simulink model "untitled"  (R2023b)
settings: Solver=VariableStepAuto  StartTime=0.0  StopTime=20  RelTol=1e-3
undefined symbols (not defined in the file): tdead, Vth
libraries: spsMosfetLib x8, spsCurrentMeasurementLib x2, spsParallelRLCBranchLib x2, simulink x2, spsLinearTransformerLib x1, spsDCVoltageSourceLib x1, slpidlib x1, spsSeriesRLCBranchLib x1, spsVoltageMeasurementLib x1, spspowerguiLib x1
settings Model: Creator=Dell  LastModifiedBy=Dell

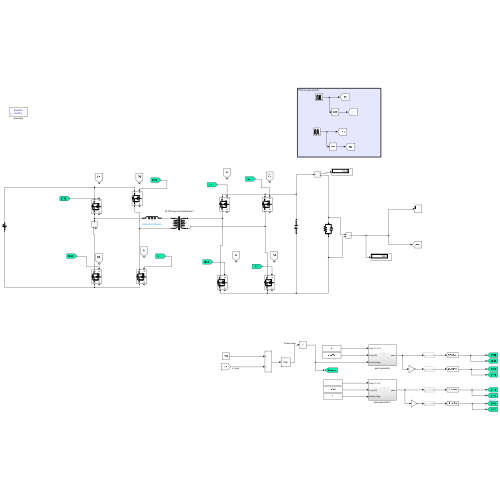
[thumbnail: Simulink's stored preview of the top-level diagram]
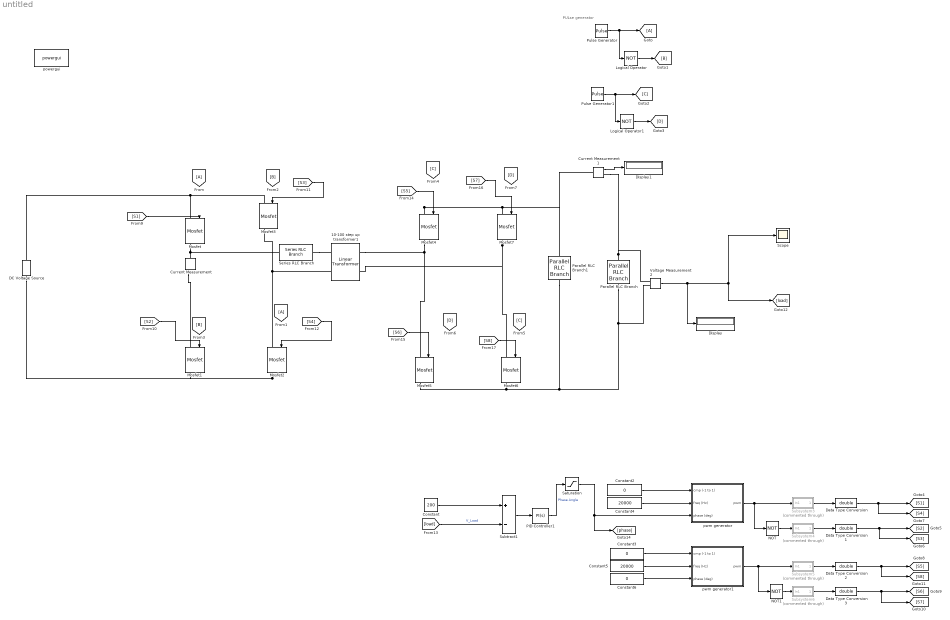
== system untitled ==
  note: PULse generator
  10-100 step up transformer1 : spsLinearTransformerLib/Linear Transformer  UNITS=pu  NominalPower=[ 2.5e3 20e3 ]  winding1="[ 400 0  0 ]"  winding2="[ 200  0  0 ]"  ThreeWindings=off  winding3=[ 315e3 0.002 0.08 ]  RmLm="[ 1e6  1e6 ]"  Measurements=None  DataType=off
  Constant : Constant  Value=200
  Constant2 : Constant  Value=0
  Constant3 : Constant  Value=0
  Constant4 : Constant  Value=20000
  Constant5 : Constant  Value=20000
  Constant6 : Constant  Value=0
  Current Measurement : spsCurrentMeasurementLib/Current Measurement  PhasorSimulation=off  OutputType=Complex  PSBequivalent=0
  Current Measurement1 : spsCurrentMeasurementLib/Current Measurement  PhasorSimulation=off  OutputType=Complex  PSBequivalent=0
  DC Voltage Source : spsDCVoltageSourceLib/DC Voltage Source  Amplitude=400  Measurements=None
  Data Type Conversion{,1..3} (4 alike) : DataTypeConversion  OutDataTypeStr=double  SaturateOnIntegerOverflow=off  RndMeth=Floor
  Display : Display
  Display1 : Display
  From : From
  From1 : From
  Goto : Goto
  Logical Operator : Logic  Operator=NOT  AllPortsSameDT=off  OutDataTypeStr=boolean
  Logical Operator1 : Logic  Operator=NOT  AllPortsSameDT=off  OutDataTypeStr=boolean
  Mosfet{,1..7} (8 alike) : spsMosfetLib/Mosfet  Ron=0.1  Lon=0  Rd=0.01  Vfd=0  IC=0  Rs=1e5  Cs=inf  Measurements=on
  NOT : Logic  Operator=NOT  IconShape=distinctive  AllPortsSameDT=off  OutDataTypeStr=boolean
  NOT1 : Logic  Operator=NOT  IconShape=distinctive  AllPortsSameDT=off  OutDataTypeStr=boolean
  PID Controller1 : slpidlib/PID Controller  Controller=PI  Form=Parallel  TimeDomain=Continuous-time  UseExternalTs=off  SampleTime=-1  IntegratorMethod=Forward Euler  FilterMethod=Forward Euler  ControllerParametersSource=internal  P=0.15  I=15  UseKiTs=off  D=0  N=100  UseFilter=on  TunerSelectOption=Transfer Function Based (PID Tuner App)  InitialConditionSource=internal  InitialConditionForIntegrator=0  InitialConditionForFilter=0  DifferentiatorICPrevScaledInput=0  ExternalReset=none  TrackingMode=off  Kt=1  LimitOutput=off  SatLimitsSource=internal  UpperSaturationLimit=inf  LowerSaturationLimit=-inf  LinearizeAsGain=on  AntiWindupMode=none  Kb=1  LimitIntegrator=off  UpperIntegratorSaturationLimit=inf  LowerIntegratorSaturationLimit=-inf  POutMin=[]  POutMax=[]  IOutMin=[]  IOutMax=[]  DOutMin=[]  DOutMax=[]  NOutMin=[]  NOutMax=[]  SumOutMin=[]  SumOutMax=[]  SaturationOutMin=[]  SaturationOutMax=[]  PParamMin=[]  PParamMax=[]  IParamMin=[]  IParamMax=[]  DParamMin=[]  DParamMax=[]  NParamMin=[]  NParamMax=[]  KbParamMin=[]  KbParamMax=[]  KtParamMin=[]  KtParamMax=[]  KbOutMin=[]  KbOutMax=[]  KtOutMin=[]  KtOutMax=[]  IntegratorOutMin=[]  IntegratorOutMax=[]  FilterOutMin=[]  FilterOutMax=[]  SumI1OutMin=[]  SumI1OutMax=[]  SumI2OutMin=[]  SumI2OutMax=[]  SumI3OutMin=[]  SumI3OutMax=[]  SumI4OutMin=[]  SumI4OutMax=[]  SumDOutMin=[]  SumDOutMax=[]  DifferentiatorOutMin=[]  DifferentiatorOutMax=[]  FilterDiffOutCoefMin=[]  FilterDiffOutCoefMax=[]  ReciprocalOutMin=[]  ReciprocalOutMax=[]  SumDenOutMin=[]  SumDenOutMax=[]  SumNumOutMin=[]  SumNumOutMax=[]  DivideOutMin=[]  DivideOutMax=[]  UdiffTsProdOutMin=[]  UdiffTsProdOutMax=[]  NTsProdOutMin=[]  NTsProdOutMax=[]  UintegralTsProdOutMin=[]  UintegralTsProdOutMax=[]  UngainTsProdOutMin=[]  UngainTsProdOutMax=[]  ClampingZeroOutDataTypeStr=Inherit: Inherit via back propagation  ClampingZeroOutMin=[]  ClampingZeroOutMax=[]  FilterDenConstantOutDataTypeStr=Inherit: Inherit via back propagation  FilterDenConstantOutMin=[]  FilterDenConstantOutMax=[]  PCopyOutDataTypeStr=Inherit: Inherit via back propagation  PCopyOutMin=[]  PCopyOutMax=[]  NCopyOutDataTypeStr=Inherit: Inherit via back propagation  NCopyOutMin=[]  NCopyOutMax=[]  IntegratorContinuousStateAttributes=''  IntegratorStateMustResolveToSignalObject=off  IntegratorRTWStateStorageClass=Auto  FilterContinuousStateAttributes=''  FilterStateMustResolveToSignalObject=off  FilterRTWStateStorageClass=Auto  ParallelPVariant=InternalParameters  IdealPVariant=Disabled  IVariant=InternalParameters  DVariant=Disabled  IntegratorVariant=Continuous  SatVariant=Disabled  AWVariant=Passthrough  PCopyVariant=Disabled  TRVariant=Disabled  FdbkBlocksVariant=Forward  IdealPFdbkVariant=Disabled  SatFdbkVariant=Disabled  DerivativeFilterVariant=Disabled  NVariant=Disabled  NCopyVariant=Disabled_SignalSpec  FilterICVariant=Disabled  IntegratorICVariant=InternalICs  ExternalResetVariant=Disabled  TRSumVariant=Passthrough  SumFdbkVariant=Disabled  SumVariant=Sum_PI  TsampFilterVariant=InternalTs  TsampNgainVariant=Passthrough  TsampIntegralVariant=Disabled_SignalSpec  ExternalSaturationOutDataTypeStr=Inherit: Same as second input
  Parallel RLC Branch : spsParallelRLCBranchLib/Parallel RLC Branch  LConnTagsString=a  RConnTagsString=__new0  BranchType=RC  Resistance=16  Inductance=1e-3  SetiL0=off  InitialCurrent=0  Capacitance=10e-6  Setx0=off  InitialVoltage=0  Measurements=None
  Parallel RLC Branch1 : spsParallelRLCBranchLib/Parallel RLC Branch  LConnTagsString=a  RConnTagsString=__new0  BranchType=C  Resistance=16  Inductance=1e-3  SetiL0=off  InitialCurrent=0  Capacitance=100e-6  Setx0=off  InitialVoltage=0  Measurements=None
  Pulse Generator : DiscretePulseGenerator  PulseType=Time based  Period=1/20e3  PulseWidth=50
  Pulse Generator1 : DiscretePulseGenerator  PulseType=Time based  Period=1/20e3  PulseWidth=50  PhaseDelay=(1/360)*(1/(20e3))
  Saturation : Saturate  UpperLimit=200  LowerLimit=0
  Scope : Scope
  Series RLC Branch : spsSeriesRLCBranchLib/Series RLC Branch  LConnTagsString=__new0  RConnTagsString=__new0  BranchType=L  Resistance=1  Inductance=0.3e-6  SetiL0=off  InitialCurrent=0  Capacitance=1e-6  Setx0=off  InitialVoltage=0  Measurements=None
  Subsystem3 : Subsystem  Commented=through
  Subsystem4 : Subsystem  Commented=through
  Subsystem5 : Subsystem  Commented=through
  Subsystem6 : Subsystem  Commented=through
  Subtract1 : Sum  Inputs=+-
  Voltage Measurement2 : spsVoltageMeasurementLib/Voltage Measurement  PhasorSimulation=off  OutputType=Complex  PSBequivalent=0
  powergui : spspowerguiLib/powergui  Priority=1  SimulationMode=Discrete  SampleTime=50e-6  frequency=60  Iterations=50  frequencyindice=0  Pbase=100e6  ErrMax=1e-4  UnitsV=kV  UnitsW=MW  buscounter=0  FunctionMessages=off  echomessages=off  EnableUseOfTLC=off  CurrentSourceSwitches=off  DisableSnubberDevices=off  DisableRonSwitches=off  DisableVfSwitches=off  DisplayEquations=off  AutomaticDiscreteSolvers=off  SolverType=Tustin/Backward Euler (TBE)  Interpol=off  ExternalGateDelay=off  methode=off  Ts=100  x0status=blocks  SPID=on  SwTol=0  HookPort=off  NonlinearTolerance=1e-4  nMaxIteration=100  ContinueOnMaxIteration=off  RestoreLinks=warning  ResistiveCurrentMeasurement=off  Frange=[0:2:500]  Ylog=off  Xlog=on  ShowGrid=off  save=off  variable=ZData  structure=0  ZoomFFT=off  StartTime=0.0  cycles=1  DisplayStyle=1  fundamental=60  FreqAxis=off  MaxFrequency=1000  frequencyindicesteady=1  RmsSteady=1  display=off
  pwm generator : Subsystem
  pwm generator1 : Subsystem
  wires:
  [S8] -> Mosfet6/1
  [S3] -> Mosfet3/1
  [S2] -> Mosfet1/1
  [S1] -> Mosfet/1
  [S7] -> Mosfet7/1
  [S5] -> Mosfet4/1
  [load] -> Subtract1/2  "V_Load"
  Current Measurement1/1 -> Display1/1
  Voltage Measurement2/1 -> Display/1, [load], Scope/1
  Pulse Generator/1 -> Logical Operator/1, Goto/1
  Pulse Generator1/1 -> [C], Logical Operator1/1
  NOT1/1 -> Subsystem6/1(In1)
  Constant2/1 -> pwm generator/1(cmp (-1 to 1))
  Constant6/1 -> pwm generator1/3(phase (deg))
  Data Type Conversion1/1 -> [S3], [S2]
  Subsystem4/1(Out1) -> Data Type Conversion1/1
  Logical Operator/1 -> [B]
  Constant3/1 -> pwm generator1/1(cmp (-1 to 1))
  Subsystem6/1(Out1) -> Data Type Conversion3/1
  pwm generator/1(pwm) -> Subsystem3/1(In1), NOT/1
  Subtract1/1 -> PID Controller1/1
  Logical Operator1/1 -> [D]
  Data Type Conversion/1 -> [S4], [S1]
  PID Controller1/1 -> Saturation/1  "Phase Angle"
  Constant5/1 -> pwm generator1/2(freq (Hz))
  Subsystem5/1(Out1) -> Data Type Conversion2/1
  [S6] -> Mosfet5/1
  NOT/1 -> Subsystem4/1(In1)
  Subsystem3/1(Out1) -> Data Type Conversion/1
  Constant/1 -> Subtract1/1
  Data Type Conversion2/1 -> [S8], [S5]
  Data Type Conversion3/1 -> [S7], [S6]
  Constant4/1 -> pwm generator/2(freq (Hz))
  [S4] -> Mosfet2/1
  pwm generator1/1(pwm) -> Subsystem5/1(In1), NOT1/1
  Saturation/1 -> [phase], pwm generator/3(phase (deg))
  connections:
  Mosfet4/LConn1 -- Parallel RLC Branch1/LConn1 -- Current Measurement1/LConn1 -- Mosfet7/LConn1
  10-100 step up transformer1/RConn1 -- Mosfet4/RConn1 -- Mosfet5/LConn1
  Voltage Measurement2/LConn2 -- Parallel RLC Branch/RConn1 -- Parallel RLC Branch1/RConn1 -- Mosfet5/RConn1 -- Mosfet6/RConn1
  10-100 step up transformer1/LConn2 -- Mosfet3/RConn1 -- Mosfet2/LConn1
  Parallel RLC Branch/LConn1 -- Voltage Measurement2/LConn1 -- Current Measurement1/RConn1
  Mosfet2/RConn1 -- Mosfet1/RConn1 -- DC Voltage Source/LConn1
  Series RLC Branch/LConn1 -- Mosfet/RConn1 -- Current Measurement/LConn1
  DC Voltage Source/RConn1 -- Mosfet/LConn1 -- Mosfet3/LConn1
  Mosfet7/RConn1 -- Mosfet6/LConn1 -- 10-100 step up transformer1/RConn2
  Current Measurement/RConn1 -- Mosfet1/LConn1
  Series RLC Branch/RConn1 -- 10-100 step up transformer1/LConn1

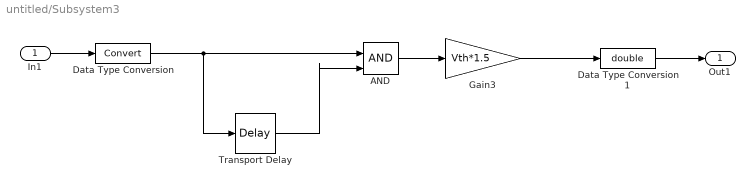
== system untitled/Subsystem3 ==
  In1 : Inport
  AND : Logic  IconShape=distinctive  AllPortsSameDT=off  OutDataTypeStr=boolean
  Data Type Conversion : DataTypeConversion  SaturateOnIntegerOverflow=off  RndMeth=Floor
  Data Type Conversion1 : DataTypeConversion  OutDataTypeStr=double  SaturateOnIntegerOverflow=off  RndMeth=Floor
  Gain3 : Gain  Gain=Vth*1.5
  Transport Delay : TransportDelay  DelayTime=tdead
  Out1 : Outport
  wires:
  Data Type Conversion/1 -> AND/1, Transport Delay/1
  In1/1 -> Data Type Conversion/1
  Transport Delay/1 -> AND/2
  AND/1 -> Gain3/1
  Gain3/1 -> Data Type Conversion1/1
  Data Type Conversion1/1 -> Out1/1

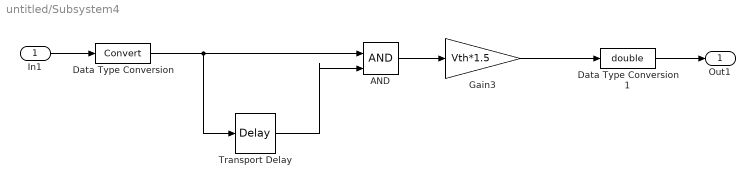
== system untitled/Subsystem4 ==
  In1 : Inport
  AND : Logic  IconShape=distinctive  AllPortsSameDT=off  OutDataTypeStr=boolean
  Data Type Conversion : DataTypeConversion  SaturateOnIntegerOverflow=off  RndMeth=Floor
  Data Type Conversion1 : DataTypeConversion  OutDataTypeStr=double  SaturateOnIntegerOverflow=off  RndMeth=Floor
  Gain3 : Gain  Gain=Vth*1.5
  Transport Delay : TransportDelay  DelayTime=tdead
  Out1 : Outport
  wires:
  Data Type Conversion1/1 -> Out1/1
  Gain3/1 -> Data Type Conversion1/1
  AND/1 -> Gain3/1
  Transport Delay/1 -> AND/2
  In1/1 -> Data Type Conversion/1
  Data Type Conversion/1 -> Transport Delay/1, AND/1

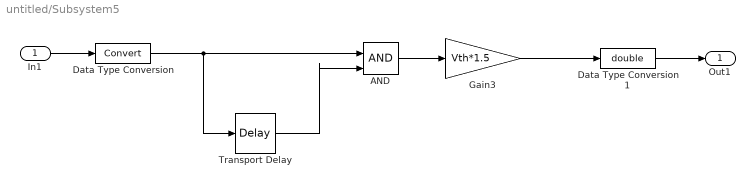
== system untitled/Subsystem5 ==
  In1 : Inport
  AND : Logic  IconShape=distinctive  AllPortsSameDT=off  OutDataTypeStr=boolean
  Data Type Conversion : DataTypeConversion  SaturateOnIntegerOverflow=off  RndMeth=Floor
  Data Type Conversion1 : DataTypeConversion  OutDataTypeStr=double  SaturateOnIntegerOverflow=off  RndMeth=Floor
  Gain3 : Gain  Gain=Vth*1.5
  Transport Delay : TransportDelay  DelayTime=tdead
  Out1 : Outport
  wires:
  Data Type Conversion/1 -> AND/1, Transport Delay/1
  In1/1 -> Data Type Conversion/1
  Transport Delay/1 -> AND/2
  AND/1 -> Gain3/1
  Gain3/1 -> Data Type Conversion1/1
  Data Type Conversion1/1 -> Out1/1

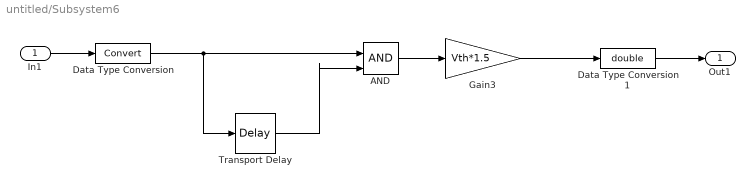
== system untitled/Subsystem6 ==
  In1 : Inport
  AND : Logic  IconShape=distinctive  AllPortsSameDT=off  OutDataTypeStr=boolean
  Data Type Conversion : DataTypeConversion  SaturateOnIntegerOverflow=off  RndMeth=Floor
  Data Type Conversion1 : DataTypeConversion  OutDataTypeStr=double  SaturateOnIntegerOverflow=off  RndMeth=Floor
  Gain3 : Gain  Gain=Vth*1.5
  Transport Delay : TransportDelay  DelayTime=tdead
  Out1 : Outport
  wires:
  Data Type Conversion1/1 -> Out1/1
  Gain3/1 -> Data Type Conversion1/1
  AND/1 -> Gain3/1
  Transport Delay/1 -> AND/2
  In1/1 -> Data Type Conversion/1
  Data Type Conversion/1 -> Transport Delay/1, AND/1

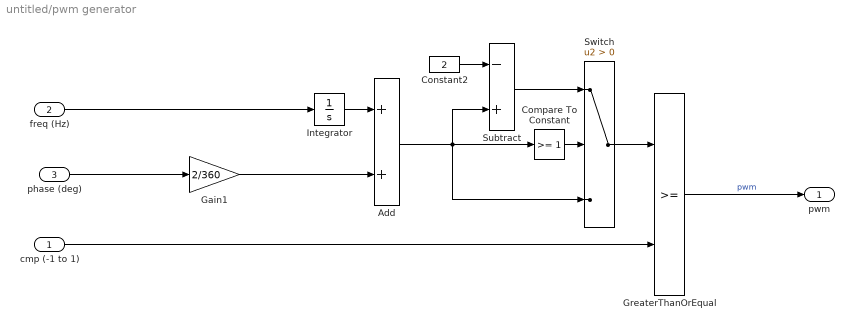
== system untitled/pwm generator ==
  cmp (-1 to 1) : Inport
  freq (Hz) : Inport  Port=2
  phase (deg) : Inport  Port=3
  Add : Sum
  Compare To Constant : simulink/Logic and Bit Operations/Compare To Constant  relop=>=  const=1  OutDataTypeStr=boolean
  Constant2 : Constant  Value=2
  Gain1 : Gain  Gain=2/360
  GreaterThanOrEqual : RelationalOperator  OutDataTypeStr=boolean  RndMeth=Simplest  InputSameDT=off
  Integrator : Integrator  WrapState=on  WrappedStateUpperValue=1  WrappedStateLowerValue=-1
  Subtract : Sum  Inputs=-+
  Switch : Switch  Criteria=u2 > Threshold  SaturateOnIntegerOverflow=off  InputSameDT=off
  pwm : Outport
  wires:
  Constant2/1 -> Subtract/1
  Gain1/1 -> Add/2
  freq (Hz)/1 -> Integrator/1
  cmp (-1 to 1)/1 -> GreaterThanOrEqual/2
  Add/1 -> Switch/3, Subtract/2, Compare To Constant/1
  Integrator/1 -> Add/1
  Compare To Constant/1 -> Switch/2
  Subtract/1 -> Switch/1
  Switch/1 -> GreaterThanOrEqual/1
  phase (deg)/1 -> Gain1/1
  GreaterThanOrEqual/1 -> pwm/1  "pwm"

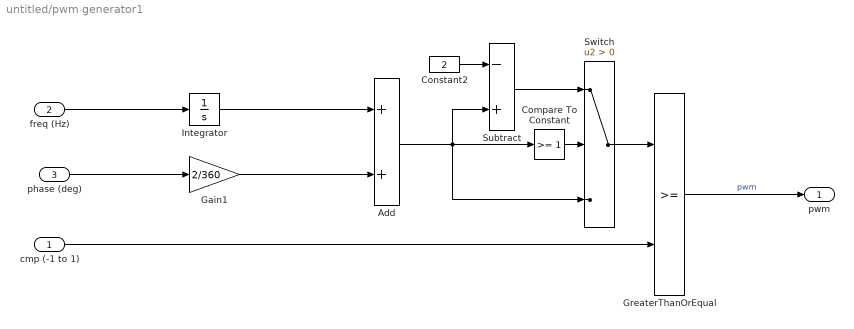
== system untitled/pwm generator1 ==
  cmp (-1 to 1) : Inport
  freq (Hz) : Inport  Port=2
  phase (deg) : Inport  Port=3
  Add : Sum
  Compare To Constant : simulink/Logic and Bit Operations/Compare To Constant  relop=>=  const=1  OutDataTypeStr=boolean
  Constant2 : Constant  Value=2
  Gain1 : Gain  Gain=2/360
  GreaterThanOrEqual : RelationalOperator  OutDataTypeStr=boolean  RndMeth=Simplest  InputSameDT=off
  Integrator : Integrator  WrapState=on  WrappedStateUpperValue=1  WrappedStateLowerValue=-1
  Subtract : Sum  Inputs=-+
  Switch : Switch  Criteria=u2 > Threshold  SaturateOnIntegerOverflow=off  InputSameDT=off
  pwm : Outport
  wires:
  GreaterThanOrEqual/1 -> pwm/1  "pwm"
  phase (deg)/1 -> Gain1/1
  Switch/1 -> GreaterThanOrEqual/1
  Subtract/1 -> Switch/1
  Compare To Constant/1 -> Switch/2
  Integrator/1 -> Add/1
  Add/1 -> Compare To Constant/1, Subtract/2, Switch/3
  cmp (-1 to 1)/1 -> GreaterThanOrEqual/2
  freq (Hz)/1 -> Integrator/1
  Gain1/1 -> Add/2
  Constant2/1 -> Subtract/1
